simulink model "thu_thap_so_lieu"  (R2016a)
settings: Solver=ode5  SolverMode=SingleTasking  StartTime=0.0  StopTime=Tstop  FixedStep=T  RelTol=1e-3
settings Model: Creator=Administrator  LastModifiedBy=Administrator
settings DebuggingCC: SFUnexpectedBacktrackingDiag=error  SFNoUnconditionalDefaultTransitionDiag=error
settings GRTTargetCC: TargetLangStandard=C99 (ISO)  GeneratePreprocessorConditionals=Use local settings
settings ConfigComp: CovMetricSettings=dwe  CovHtmlReporting=off  CovSaveCumulativeToWorkspaceVar=off  CovSaveSingleToWorkspaceVar=off  CovExternalEMLEnable=on

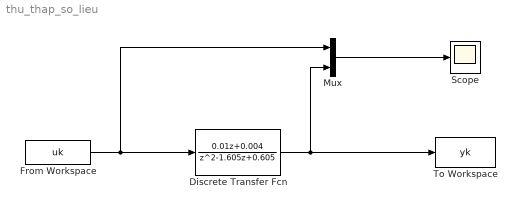
== system thu_thap_so_lieu ==
  Discrete Transfer Fcn : DiscreteTransferFcn  Numerator=[0.01 0.004]  Denominator=[1 -1.605 0.605]  SampleTime=0.01
  From Workspace : FromWorkspace  VariableName=uk  OutDataTypeStr=double  SampleTime=0.01
  Mux : Mux  Inputs=2
  Scope : Scope
  To Workspace : ToWorkspace  VariableName=yk  SampleTime=0.01
  wires:
  Mux/1 -> Scope/1
  Discrete Transfer Fcn/1 -> To Workspace/1, Mux/2
  From Workspace/1 -> Mux/1, Discrete Transfer Fcn/1
